simulink model "CTRL_TRGT_test"  (R2023b)
settings: Solver=FixedStepAuto  StartTime=0.0  StopTime=10.0  FixedStep=0.01  RelTol=1e-3
libraries: CTRL_TRGT x1, simulink x1
settings Model: Creator=blatak  LastModifiedBy=blatak

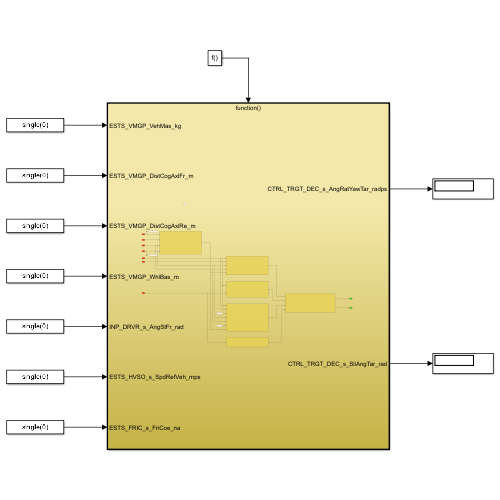
[thumbnail: Simulink's stored preview of the top-level diagram]
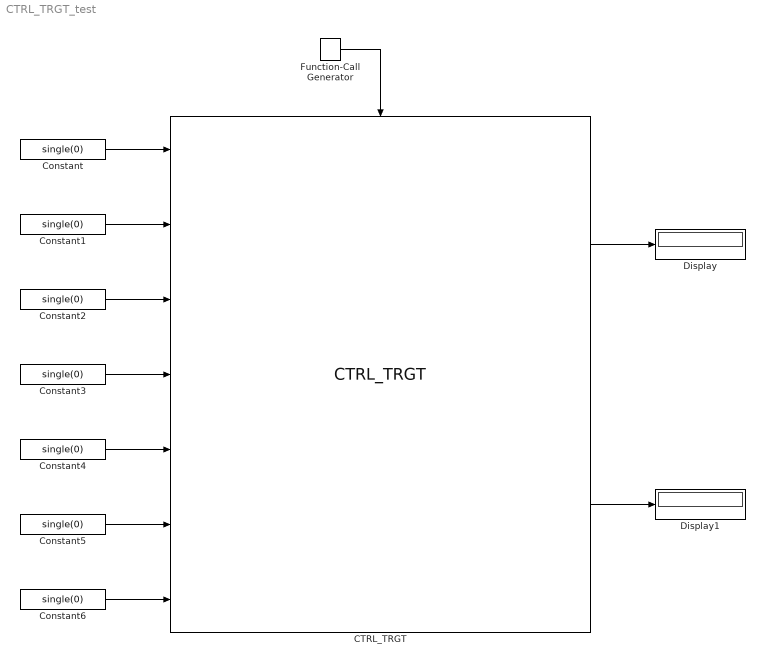
== system CTRL_TRGT_test ==
  CTRL_TRGT : CTRL_TRGT/CTRL_TRGT  SystemSampleTime=-1  VariantActivationTime=update diagram  AllowFlexibleInterface=on  Latency=0  AutoFrameSizeCalculation=off
  Constant{,1..6} (7 alike) : Constant  Value=single(0)  OutDataTypeStr=single
  Display : Display
  Display1 : Display
  Function-Call Generator : simulink/Ports & Subsystems/Function-Call Generator  sample_time=0.01  numberOfIterations=1  DisallowWideOutput=off
  wires:
  Constant/1 -> CTRL_TRGT/1
  Constant1/1 -> CTRL_TRGT/2
  Constant2/1 -> CTRL_TRGT/3
  Constant3/1 -> CTRL_TRGT/4
  Constant4/1 -> CTRL_TRGT/5
  Constant5/1 -> CTRL_TRGT/6
  Constant6/1 -> CTRL_TRGT/7
  CTRL_TRGT/1 -> Display/1
  CTRL_TRGT/2 -> Display1/1
  Function-Call Generator/1 -> CTRL_TRGT/Trigger
